simulink model "Multilevel_inverter_PD"  (R2022a)
settings: Solver=FixedStepDiscrete  StartTime=0.0  StopTime=3  RelTol=1e-3
libraries: spsMosfetLib x36, spsDCVoltageSourceLib x9, simulink x9, spsGroundLib x3, spsPermanentMagnetSynchronousMachineLib x1, spsThreePhaseVIMeasurementLib x1, spspowerguiLib x1
settings Model: Creator=Admin  LastModifiedBy=Admin
settings OptimizationCC: UseDivisionForNetSlopeComputation=UseDivisionForReciprocalsOfIntegersOnly  DefaultUnderspecifiedDataType=single
settings DebuggingCC: SignalInfNanChecking=warning  ReadBeforeWriteMsg=DisableAll  WriteAfterWriteMsg=DisableAll  WriteAfterReadMsg=DisableAll  UniqueDataStoreMsg=error  AssertControl=DisableAll  SFUndirectedBroadcastEventsDiag=error
settings ModelReferenceCC: UpdateModelReferenceTargets=IfOutOfDate
settings SFSimCC: SFSimEcho=off  SimIntegrity=off  CompileTimeRecursionLimit=0
settings ConfigComp: CovScope=ReferencedModels

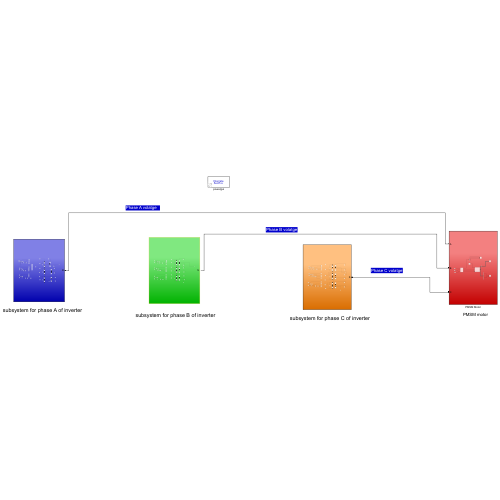
[thumbnail: Simulink's stored preview of the top-level diagram]
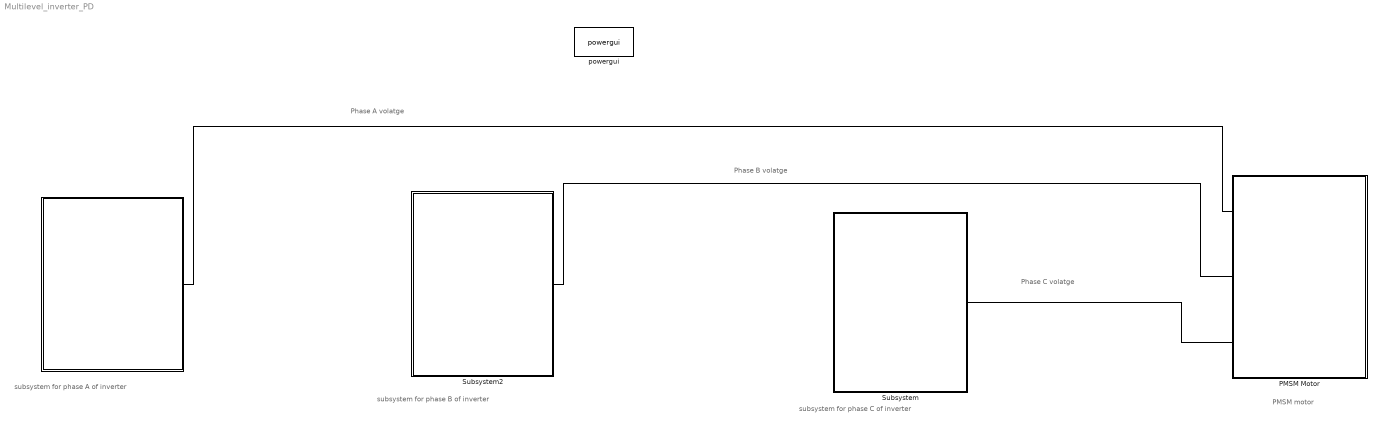
== system Multilevel_inverter_PD ==
  note: Phase A volatge
  note: PMSM motor
  note: subsystem for phase A of inverter
  note: subsystem for phase B of inverter
  note: subsystem for phase C of inverter
  note: Phase B volatge
  note: Phase C volatge
  "  " : Subsystem
  PMSM Motor : Subsystem
  Subsystem : Subsystem
  Subsystem2 : Subsystem
  powergui : spspowerguiLib/powergui  Priority=1  SimulationMode=Discrete  SampleTime=50e-6  frequency=60  Iterations=50  frequencyindice=0  Pbase=100e6  ErrMax=1e-4  UnitsV=kV  UnitsW=MW  buscounter=0  FunctionMessages=off  echomessages=off  EnableUseOfTLC=off  CurrentSourceSwitches=off  DisableSnubberDevices=off  DisableRonSwitches=off  DisableVfSwitches=off  DisplayEquations=off  AutomaticDiscreteSolvers=off  SolverType=Tustin/Backward Euler (TBE)  Interpol=off  ExternalGateDelay=off  methode=off  Ts=100  x0status=blocks  SPID=off  SwTol=0  HookPort=off  NonlinearTolerance=1e-4  nMaxIteration=100  ContinueOnMaxIteration=off  RestoreLinks=warning  ResistiveCurrentMeasurement=off  Frange=[0:2:500]  Ylog=off  Xlog=on  ShowGrid=off  save=off  variable=ZData  structure=0  ZoomFFT=off  StartTime=0.0  cycles=1  DisplayStyle=1  fundamental=60  FreqAxis=off  MaxFrequency=1000  frequencyindicesteady=1  RmsSteady=1  display=off
  connections:
  PMSM Motor/LConn1 -- "  "/RConn1
  PMSM Motor/LConn2 -- Subsystem2/RConn1
  Subsystem/RConn1 -- PMSM Motor/LConn3

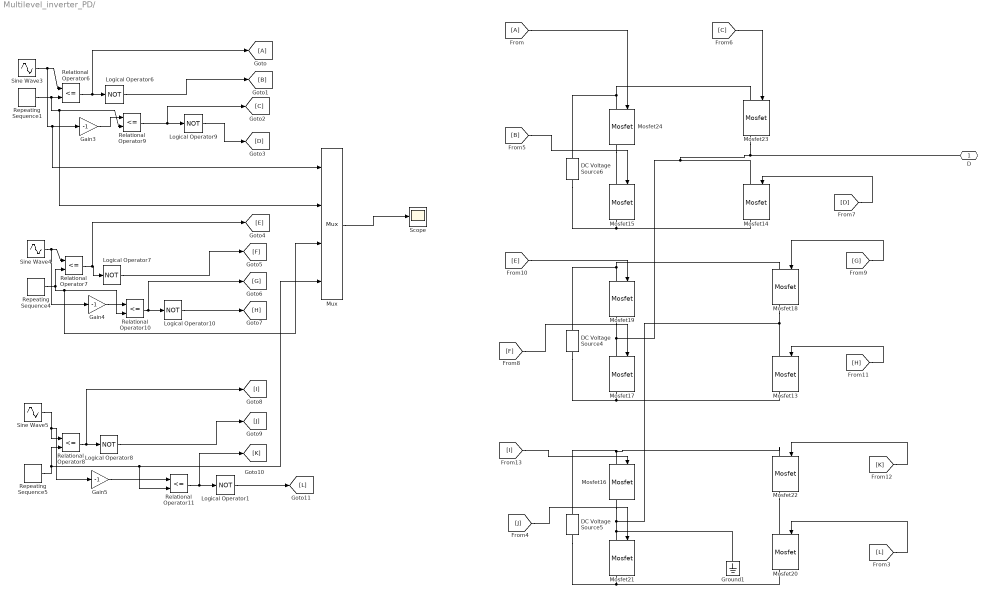
== system Multilevel_inverter_PD/   ==
  DC Voltage Source4 : spsDCVoltageSourceLib/DC Voltage Source  Amplitude=100  Measurements=None
  DC Voltage Source5 : spsDCVoltageSourceLib/DC Voltage Source  Amplitude=100  Measurements=None
  DC Voltage Source6 : spsDCVoltageSourceLib/DC Voltage Source  Amplitude=100  Measurements=None
  From : From
  Gain3 : Gain  Gain=-1
  Gain4 : Gain  Gain=-1
  Gain5 : Gain  Gain=-1
  Goto : Goto
  Ground1 : spsGroundLib/Ground  LConnTagsString=a
  Logical Operator{1,6..10} (6 alike) : Logic  Operator=NOT  AllPortsSameDT=off  OutDataTypeStr=boolean
  Mosfet{13..24} (12 alike) : spsMosfetLib/Mosfet  Ron=0.1  Lon=0  Rd=0.01  Vfd=0  IC=0  Rs=1e5  Cs=inf  Measurements=on
  Mux : Mux
  Relational Operator{6..11} (6 alike) : RelationalOperator  Operator=<=  OutDataTypeStr=boolean  RndMeth=Simplest  InputSameDT=off
  Repeating Sequence1 : simulink/Sources/Repeating Sequence  rep_seq_t=[0 0.5 1]/1000  rep_seq_y=[0 1 0]
  Repeating Sequence4 : simulink/Sources/Repeating Sequence  rep_seq_t=[0 0.5 1]/1000  rep_seq_y=[1 2 1]
  Repeating Sequence5 : simulink/Sources/Repeating Sequence  rep_seq_t=[0 0.5 1]/1000  rep_seq_y=[0 -1 0]
  Scope : Scope
  Sine Wave3 : Sin  Amplitude=3  Frequency=314.15  SampleTime=0
  Sine Wave4 : Sin  Amplitude=3  Frequency=2*pi*50  SampleTime=0
  Sine Wave5 : Sin  Amplitude=3  Frequency=2*pi*50  SampleTime=0
  D : PMIOPort  Side=Right
  wires:
  Gain3/1 -> Relational Operator9/1
  Repeating Sequence4/1 -> Relational Operator7/2, Mux/3, Relational Operator10/2
  Sine Wave5/1 -> Gain5/1, Relational Operator8/1
  Gain5/1 -> Relational Operator11/1
  Relational Operator10/1 -> [G], Logical Operator10/1
  Gain4/1 -> Relational Operator10/1
  Relational Operator6/1 -> Goto/1, Logical Operator6/1
  Repeating Sequence1/1 -> Mux/2, Relational Operator9/2, Relational Operator6/2
  Repeating Sequence5/1 -> Mux/4, Relational Operator11/2, Relational Operator8/2
  Sine Wave4/1 -> Gain4/1, Relational Operator7/1
  Relational Operator7/1 -> [E], Logical Operator7/1
  Relational Operator9/1 -> [C], Logical Operator9/1
  Sine Wave3/1 -> Mux/1, Gain3/1, Relational Operator6/1
  Relational Operator8/1 -> [I], Logical Operator8/1
  From/1 -> Mosfet24/1
  Logical Operator6/1 -> [B]
  Logical Operator9/1 -> [D]
  Logical Operator7/1 -> [F]
  Logical Operator10/1 -> [H]
  Logical Operator8/1 -> [J]
  [B] -> Mosfet15/1
  [C] -> Mosfet23/1
  [D] -> Mosfet14/1
  [E] -> Mosfet19/1
  [G] -> Mosfet18/1
  [F] -> Mosfet17/1
  [H] -> Mosfet13/1
  [I] -> Mosfet16/1
  [K] -> Mosfet22/1
  [L] -> Mosfet20/1
  [J] -> Mosfet21/1
  Mux/1 -> Scope/1
  Relational Operator11/1 -> [K], Logical Operator1/1
  Logical Operator1/1 -> [L]
  connections:
  Mosfet14/RConn1 -- DC Voltage Source6/LConn1 -- Mosfet15/RConn1
  Mosfet19/RConn1 -- Mosfet17/LConn1 -- Mosfet23/RConn1 -- D/RConn1 -- Mosfet14/LConn1
  DC Voltage Source6/RConn1 -- Mosfet23/LConn1 -- Mosfet24/LConn1
  DC Voltage Source4/RConn1 -- Mosfet18/LConn1 -- Mosfet19/LConn1
  Mosfet21/LConn1 -- Ground1/LConn1 -- Mosfet18/RConn1 -- Mosfet13/LConn1 -- Mosfet16/RConn1
  Mosfet24/RConn1 -- Mosfet15/LConn1
  Mosfet13/RConn1 -- DC Voltage Source4/LConn1 -- Mosfet17/RConn1
  Mosfet20/RConn1 -- DC Voltage Source5/LConn1 -- Mosfet21/RConn1
  Mosfet22/LConn1 -- DC Voltage Source5/RConn1 -- Mosfet16/LConn1
  Mosfet22/RConn1 -- Mosfet20/LConn1

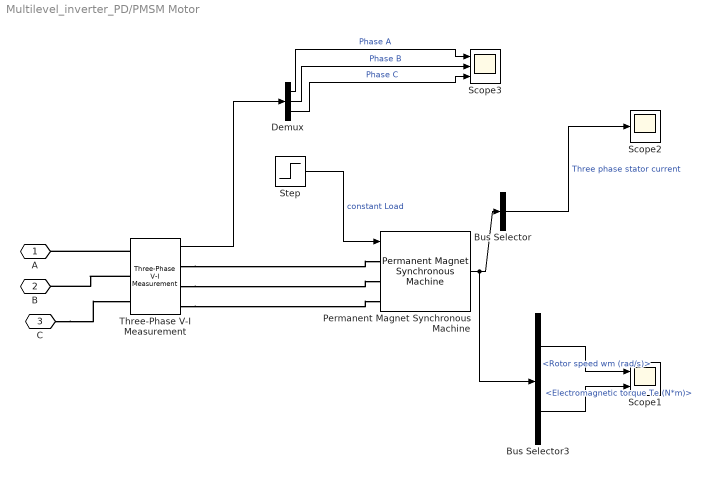
== system Multilevel_inverter_PD/PMSM Motor ==
  Bus Selector : BusSelector  OutputSignals=Stator current is_a (A),Stator current is_b (A),Stator current is_c (A)  OutputAsBus=on
  Bus Selector3 : BusSelector  OutputSignals=Rotor speed wm (rad/s),Electromagnetic torque Te (N*m)
  Demux : Demux  Outputs=3
  Permanent Magnet Synchronous Machine : spsPermanentMagnetSynchronousMachineLib/Permanent Magnet Synchronous Machine  NbPhases=3  FluxDistribution=Sinusoidal  RotorType=Round  MechanicalLoad=Torque Tm  PresetModel="02:  1.7 Nm 300 Vdc 3750 RPM - 1.7 Nm"  ShowDetailedParameters=on  MeasurementBus=off  Resistance=4.765  Inductance=8.5e-3  dqInductances=[8.5e-3,8.5e-3]  La=0.014  MachineConstant=Flux linkage established by magnets (V.s)  Flux=0.1848  VoltageCst=67.038  TorqueCst=0.5544  Flat=120  Mechanical=[0.0001051 4.047e-05 2 0]  PolePairs=2  InitialConditions=[0,0, 0,0]  InitialConditions5ph=[0 0 0 0 0 0]  RefAngle=90 degrees behind phase A axis (modified Park)  IterativeDiscreteModel=Trapezoidal non iterative  TsBlock=-1  TsPowergui=0
      link override Electrical model/iq,id/iq/Discrete-Time Integrator: InitialCondition=PM.isdo
  Scope1 : Scope  NumInputPorts=2
  Scope2 : Scope
  Scope3 : Scope  NumInputPorts=3
  Step : Step  Time=0.2  Before=1  After=3  SampleTime=0
  Three-Phase V-I Measurement : spsThreePhaseVIMeasurementLib/Three-Phase V-I Measurement  VoltageMeasurement=phase-to-phase  SetLabelV=off  LabelV=Vabc  Vpu=off  VpuLL=off  CurrentMeasurement=no  SetLabelI=off  LabelI=Iabc  Ipu=off  Pbase=100e6  Vbase=500e3  OutputType=Complex  PhasorSimulation=off  PSBequivalent=0
  A : PMIOPort  Side=Left
  B : PMIOPort  Port=2  Side=Left
  C : PMIOPort  Port=3  Side=Left
  wires:
  Demux/3 -> Scope3/3  "Phase C"
  Permanent Magnet Synchronous Machine/1 -> Bus Selector3/1, Bus Selector/1
  Demux/1 -> Scope3/1  "Phase A"
  Step/1 -> Permanent Magnet Synchronous Machine/1  "constant Load"
  Three-Phase V-I Measurement/1 -> Demux/1
  Demux/2 -> Scope3/2  "Phase B"
  Bus Selector/1 -> Scope2/1  "Three phase stator current"
  Bus Selector3/1 -> Scope1/1  "<Rotor speed wm (rad/s)>"
  Bus Selector3/2 -> Scope1/2  "<Electromagnetic torque Te (N*m)>"
  connections:
  Three-Phase V-I Measurement/RConn2 -- Permanent Magnet Synchronous Machine/LConn2
  Three-Phase V-I Measurement/RConn1 -- Permanent Magnet Synchronous Machine/LConn1
  Three-Phase V-I Measurement/RConn3 -- Permanent Magnet Synchronous Machine/LConn3
  Three-Phase V-I Measurement/LConn2 -- B/RConn1
  Three-Phase V-I Measurement/LConn1 -- A/RConn1
  C/RConn1 -- Three-Phase V-I Measurement/LConn3

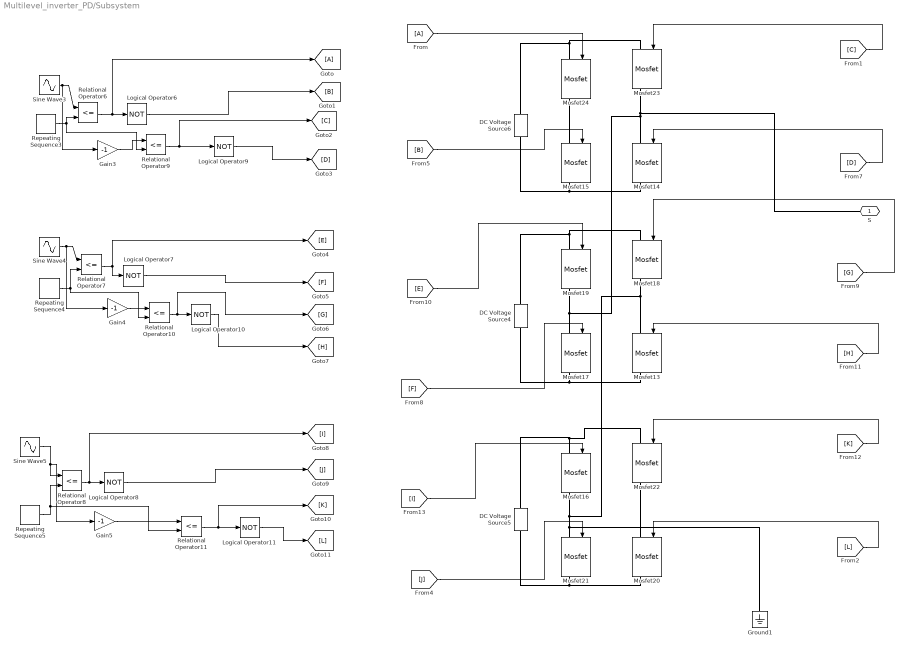
== system Multilevel_inverter_PD/Subsystem ==
  DC Voltage Source4 : spsDCVoltageSourceLib/DC Voltage Source  Amplitude=200  Measurements=None
  DC Voltage Source5 : spsDCVoltageSourceLib/DC Voltage Source  Amplitude=200  Measurements=None
  DC Voltage Source6 : spsDCVoltageSourceLib/DC Voltage Source  Amplitude=200  Measurements=None
  From : From
  Gain3 : Gain  Gain=-1
  Gain4 : Gain  Gain=-1
  Gain5 : Gain  Gain=-1
  Goto : Goto
  Ground1 : spsGroundLib/Ground  LConnTagsString=a
  Logical Operator{6..11} (6 alike) : Logic  Operator=NOT  AllPortsSameDT=off  OutDataTypeStr=boolean
  Mosfet{13..24} (12 alike) : spsMosfetLib/Mosfet  Ron=0.1  Lon=0  Rd=0.01  Vfd=0  IC=0  Rs=1e5  Cs=inf  Measurements=on
  Relational Operator{6..11} (6 alike) : RelationalOperator  Operator=<=  OutDataTypeStr=boolean  RndMeth=Simplest  InputSameDT=off
  Repeating Sequence3 : simulink/Sources/Repeating Sequence  rep_seq_t=[0 0.5 1]/1000  rep_seq_y=[0 1 0]
  Repeating Sequence4 : simulink/Sources/Repeating Sequence  rep_seq_t=[0 0.5 1]/1000  rep_seq_y=[1 2 1]
  Repeating Sequence5 : simulink/Sources/Repeating Sequence  rep_seq_t=[0 0.5 1]/1000  rep_seq_y=[0 -1 0]
  Sine Wave3 : Sin  Amplitude=3  Frequency=314.15  Phase=(4*pi)/3  SampleTime=0
  Sine Wave4 : Sin  Amplitude=3  Frequency=2*pi*50  Phase=(4*pi)/3  SampleTime=0
  Sine Wave5 : Sin  Amplitude=3  Frequency=2*pi*50  Phase=(4*pi)/3  SampleTime=0
  S : PMIOPort  Side=Right
  wires:
  Relational Operator8/1 -> [I], Logical Operator8/1
  Sine Wave3/1 -> Gain3/1, Relational Operator6/1
  Relational Operator10/1 -> [G], Logical Operator10/1
  Gain4/1 -> Relational Operator10/1
  Repeating Sequence4/1 -> Relational Operator7/2, Relational Operator10/2
  Relational Operator11/1 -> [K], Logical Operator11/1
  Relational Operator7/1 -> Logical Operator7/1, [E]
  Sine Wave4/1 -> Gain4/1, Relational Operator7/1
  Repeating Sequence3/1 -> Relational Operator6/2, Relational Operator9/2
  Repeating Sequence5/1 -> Relational Operator11/2, Relational Operator8/2
  Sine Wave5/1 -> Gain5/1, Relational Operator8/1
  Relational Operator9/1 -> [C], Logical Operator9/1
  Gain3/1 -> Relational Operator9/1
  Relational Operator6/1 -> Goto/1, Logical Operator6/1
  Gain5/1 -> Relational Operator11/1
  Logical Operator6/1 -> [B]
  Logical Operator9/1 -> [D]
  Logical Operator7/1 -> [F]
  Logical Operator10/1 -> [H]
  Logical Operator8/1 -> [J]
  Logical Operator11/1 -> [L]
  [C] -> Mosfet23/1
  [D] -> Mosfet14/1
  [G] -> Mosfet18/1
  [H] -> Mosfet13/1
  [K] -> Mosfet22/1
  [L] -> Mosfet20/1
  From/1 -> Mosfet24/1
  [B] -> Mosfet15/1
  [E] -> Mosfet19/1
  [F] -> Mosfet17/1
  [I] -> Mosfet16/1
  [J] -> Mosfet21/1
  connections:
  Mosfet20/RConn1 -- DC Voltage Source5/LConn1 -- Mosfet21/RConn1
  Mosfet13/LConn1 -- Mosfet16/RConn1 -- Ground1/LConn1 -- Mosfet21/LConn1 -- Mosfet18/RConn1
  Mosfet22/LConn1 -- DC Voltage Source5/RConn1 -- Mosfet16/LConn1
  Mosfet22/RConn1 -- Mosfet20/LConn1
  Mosfet13/RConn1 -- DC Voltage Source4/LConn1 -- Mosfet17/RConn1
  DC Voltage Source4/RConn1 -- Mosfet18/LConn1 -- Mosfet19/LConn1
  Mosfet24/RConn1 -- Mosfet15/LConn1
  Mosfet19/RConn1 -- Mosfet23/RConn1 -- S/RConn1 -- Mosfet14/LConn1 -- Mosfet17/LConn1
  Mosfet14/RConn1 -- DC Voltage Source6/LConn1 -- Mosfet15/RConn1
  DC Voltage Source6/RConn1 -- Mosfet23/LConn1 -- Mosfet24/LConn1

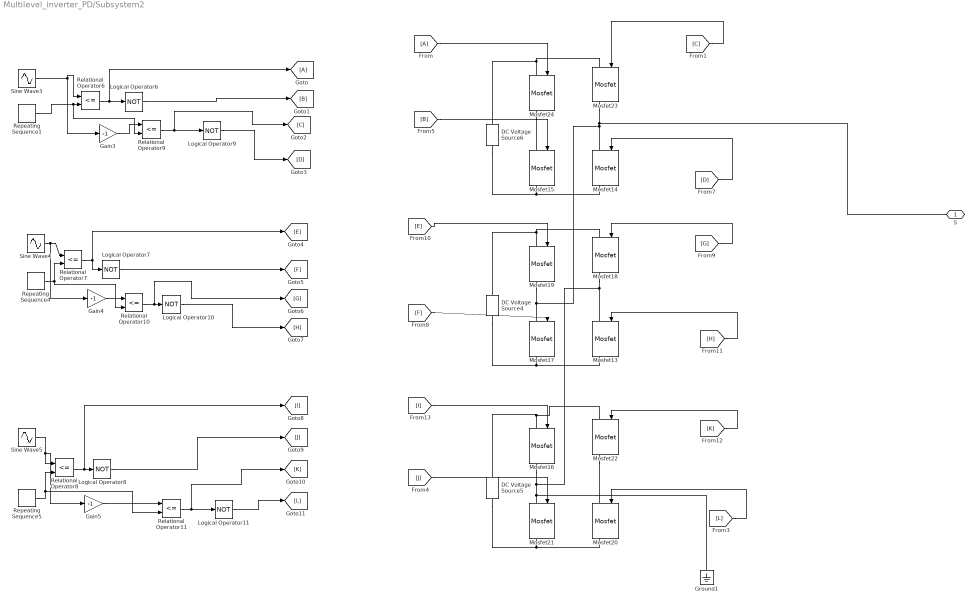
== system Multilevel_inverter_PD/Subsystem2 ==
  DC Voltage Source4 : spsDCVoltageSourceLib/DC Voltage Source  Amplitude=200  Measurements=None
  DC Voltage Source5 : spsDCVoltageSourceLib/DC Voltage Source  Amplitude=200  Measurements=None
  DC Voltage Source6 : spsDCVoltageSourceLib/DC Voltage Source  Amplitude=200  Measurements=None
  From : From
  Gain3 : Gain  Gain=-1
  Gain4 : Gain  Gain=-1
  Gain5 : Gain  Gain=-1
  Goto : Goto
  Ground1 : spsGroundLib/Ground  LConnTagsString=a
  Logical Operator{6..11} (6 alike) : Logic  Operator=NOT  AllPortsSameDT=off  OutDataTypeStr=boolean
  Mosfet{13..24} (12 alike) : spsMosfetLib/Mosfet  Ron=0.1  Lon=0  Rd=0.01  Vfd=0  IC=0  Rs=1e5  Cs=inf  Measurements=on
  Relational Operator{6..11} (6 alike) : RelationalOperator  Operator=<=  OutDataTypeStr=boolean  RndMeth=Simplest  InputSameDT=off
  Repeating Sequence1 : simulink/Sources/Repeating Sequence  rep_seq_t=[0 0.5 1]/1000  rep_seq_y=[0 1 0]
  Repeating Sequence4 : simulink/Sources/Repeating Sequence  rep_seq_t=[0 0.5 1]/1000  rep_seq_y=[1 2 1]
  Repeating Sequence5 : simulink/Sources/Repeating Sequence  rep_seq_t=[0 0.5 1]/1000  rep_seq_y=[0 -1 0]
  Sine Wave3 : Sin  Amplitude=3  Frequency=314.15  Phase=(2*pi)/3  SampleTime=0
  Sine Wave4 : Sin  Amplitude=3  Frequency=2*pi*50  Phase=(2*pi)/3  SampleTime=0
  Sine Wave5 : Sin  Amplitude=3  Frequency=2*pi*50  Phase=(2*pi)/3  SampleTime=0
  S : PMIOPort  Side=Right
  wires:
  Sine Wave4/1 -> Gain4/1, Relational Operator7/1
  Sine Wave3/1 -> Relational Operator6/1, Gain3/1
  Relational Operator6/1 -> Goto/1, Logical Operator6/1
  Relational Operator7/1 -> Logical Operator7/1, [E]
  Sine Wave5/1 -> Gain5/1, Relational Operator8/1
  Gain3/1 -> Relational Operator9/1
  Repeating Sequence4/1 -> Relational Operator7/2, Relational Operator10/2
  Relational Operator11/1 -> [K], Logical Operator11/1
  Relational Operator10/1 -> [G], Logical Operator10/1
  Gain4/1 -> Relational Operator10/1
  Repeating Sequence5/1 -> Relational Operator11/2, Relational Operator8/2
  Gain5/1 -> Relational Operator11/1
  Relational Operator9/1 -> [C], Logical Operator9/1
  Relational Operator8/1 -> [I], Logical Operator8/1
  Logical Operator6/1 -> [B]
  Logical Operator9/1 -> [D]
  Logical Operator7/1 -> [F]
  Logical Operator10/1 -> [H]
  Logical Operator8/1 -> [J]
  Logical Operator11/1 -> [L]
  From/1 -> Mosfet24/1
  [B] -> Mosfet15/1
  [E] -> Mosfet19/1
  [F] -> Mosfet17/1
  [I] -> Mosfet16/1
  [J] -> Mosfet21/1
  [D] -> Mosfet14/1
  [G] -> Mosfet18/1
  [H] -> Mosfet13/1
  [K] -> Mosfet22/1
  [L] -> Mosfet20/1
  [C] -> Mosfet23/1
  Repeating Sequence1/1 -> Relational Operator9/2, Relational Operator6/2
  connections:
  Mosfet19/RConn1 -- Mosfet17/LConn1 -- Mosfet23/RConn1 -- S/RConn1 -- Mosfet14/LConn1
  Mosfet17/RConn1 -- Mosfet13/RConn1 -- DC Voltage Source4/LConn1
  Mosfet13/LConn1 -- Mosfet18/RConn1 -- Mosfet16/RConn1 -- Ground1/LConn1 -- Mosfet21/LConn1
  Mosfet24/LConn1 -- DC Voltage Source6/RConn1 -- Mosfet23/LConn1
  Mosfet24/RConn1 -- Mosfet15/LConn1
  Mosfet21/RConn1 -- Mosfet20/RConn1 -- DC Voltage Source5/LConn1
  Mosfet16/LConn1 -- Mosfet22/LConn1 -- DC Voltage Source5/RConn1
  Mosfet19/LConn1 -- DC Voltage Source4/RConn1 -- Mosfet18/LConn1
  Mosfet15/RConn1 -- Mosfet14/RConn1 -- DC Voltage Source6/LConn1
  Mosfet22/RConn1 -- Mosfet20/LConn1
